simulink model "H036_Boost_Converter"  (R2021a)
settings: Solver=VariableStepAuto  StartTime=0.0  StopTime=10.0  RelTol=1e-3
undefined symbols (not defined in the file): K
settings Model: Creator=Pallavi  LastModifiedBy=Pallavi

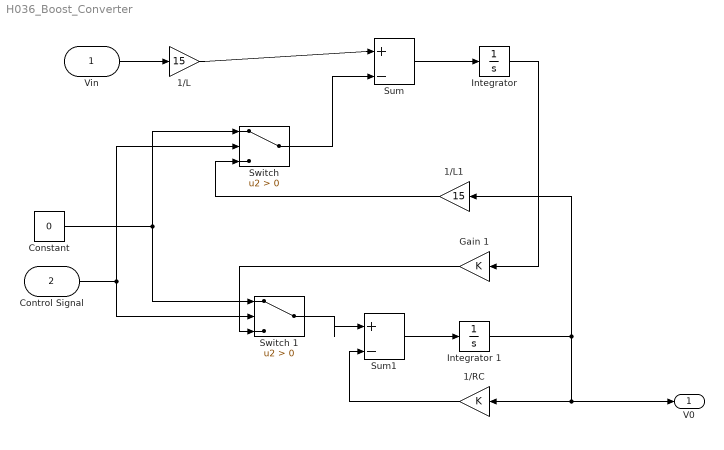
== system H036_Boost_Converter ==
  Vin : Inport
  Control Signal : Inport  Port=2
  1/L : Gain  Gain=15
  1/L1 : Gain  Gain=15
  1/RC : Gain  Gain=K
  "Constant " : Constant  Value=0
  Gain 1 : Gain  Gain=K
  "Integrator " : Integrator
  Integrator 1 : Integrator
  Sum : Sum  Inputs=|+-
  Sum1 : Sum  Inputs=|+-
  "Switch " : Switch  Criteria=u2 > Threshold
  Switch 1 : Switch  Criteria=u2 > Threshold
  V0 : Outport
  wires:
  Vin/1 -> 1/L/1
  1/L/1 -> Sum/1
  Sum/1 -> "Integrator "/1
  "Switch "/1 -> Sum/2
  "Integrator "/1 -> Gain 1/1
  Gain 1/1 -> Switch 1/3
  "Constant "/1 -> Switch 1/1, "Switch "/1
  Control Signal/1 -> Switch 1/2, "Switch "/2
  1/L1/1 -> "Switch "/3
  Integrator 1/1 -> 1/RC/1, V0/1, 1/L1/1
  Switch 1/1 -> Sum1/1
  1/RC/1 -> Sum1/2
  Sum1/1 -> Integrator 1/1
